simulink model "inter_machine_oscillation"  (R2014a)
settings: Solver=ode23tb  StartTime=0.0  StopTime=10  MaxStep=1/60  RelTol=1e-4
StartFcn:
  | tic;
StopFcn:
  | toc;
libraries: powerlib x6, simulink x2
settings Model: Creator=gdudgeon  LastModifiedBy=cosorio
settings DataIOCC: SaveOutput=off  DSMLogging=off  SaveTime=off
settings OptimizationCC: ExpressionDepthLimit=2147483647
settings DebuggingCC: UnderspecifiedInitializationDetection=Classic  FcnCallInpInsideContextMsg=UseLocalSettings  StateNameClashWarn=warning
settings GRTTargetCC: CombineOutputUpdateFcns=off  GRTInterface=on

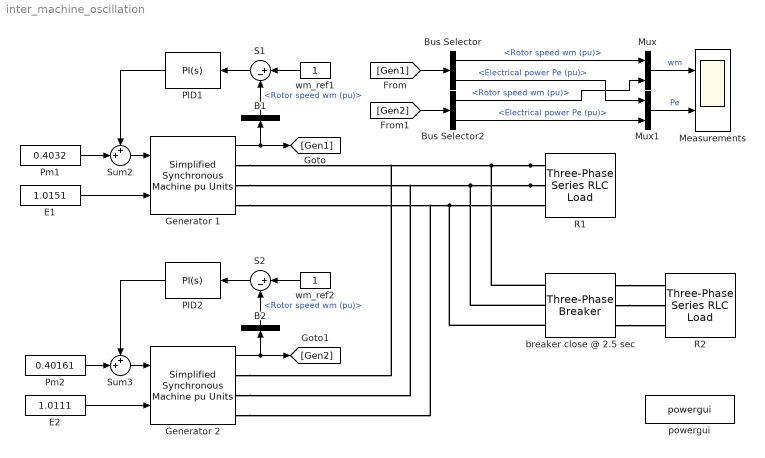
== system inter_machine_oscillation ==
  B1 : BusSelector  OutputSignals=Rotor speed wm (pu)
  B2 : BusSelector  OutputSignals=Rotor speed wm (pu)
  Bus Selector : BusSelector  OutputSignals=Rotor speed wm (pu),Electrical power Pe (pu)
  Bus Selector2 : BusSelector  OutputSignals=Rotor speed wm (pu),Electrical power Pe (pu)
  E1 : Constant  Value=1.0151
  E2 : Constant  Value=1.0111
  Generator 1 : powerlib/Machines/Simplified Synchronous Machine pu Units  ConnectionType=3-wire Y  MechanicalLoad=Mechanical power Pm  MeasurementBus=off  NominalParameters=[5e6 6600 60]  Mechanical=[3.7 0 20]  InternalRL="[0.02  0.3]"  InitialConditions=[0 6.78897 0.4 0.4 0.4 0 -120 120]  Units=0  LoadFlowParameters=[1 2000040 0 0 0]  TsPowergui=0  TsBlock=-1  BusType=PQ  Pref=2e6  Qref=0  Qmin=-inf  Qmax=+inf  PLF=0  QLF=0
      settings: AttributesFormatString=%<NominalParameters>
  Generator 2 : powerlib/Machines/Simplified Synchronous Machine pu Units  ConnectionType=3-wire Y  MechanicalLoad=Mechanical power Pm  MeasurementBus=off  NominalParameters=[5e6 6600 60]  Mechanical=[1.7 0 20]  InternalRL="[0.01  0.3]"  InitialConditions=[0 6.81591 0.400009 0.400009 0.400009 1.20401e-12 -120 120]  Units=0  LoadFlowParameters=[2 2000000 0 0 0]  TsPowergui=0  TsBlock=-1  BusType=swing  Pref=0  Qref=0  Qmin=-inf  Qmax=+inf  PLF=0  QLF=0
      settings: AttributesFormatString=%<NominalParameters>
  Measurements : Scope  NumInputPorts=2
      settings: YMin=0.8~0.25  YMax=1.1~0.75  SaveName=measurements
  Mux : Mux  Inputs=2
  Mux1 : Mux  Inputs=2
  PID1 : simulink/Continuous/PID Controller  Controller=PI  TimeDomain=Continuous-time  SampleTime=1  IntegratorMethod=Forward Euler  FilterMethod=Forward Euler  Form=Parallel  P=25  I=50  D=0  N=100  InitialConditionSource=internal  InitialConditionForIntegrator=0  InitialConditionForFilter=0  ExternalReset=none  LimitOutput=off  UpperSaturationLimit=2  LowerSaturationLimit=0  LinearizeAsGain=on  AntiWindupMode=none  Kb=1  TrackingMode=off  Kt=1  PParamMin=[]  PParamMax=[]  IParamMin=[]  IParamMax=[]  DParamMin=[]  DParamMax=[]  NParamMin=[]  NParamMax=[]  KbParamMin=[]  KbParamMax=[]  KtParamMin=[]  KtParamMax=[]  POutMin=[]  POutMax=[]  IOutMin=[]  IOutMax=[]  DOutMin=[]  DOutMax=[]  NOutMin=[]  NOutMax=[]  KbOutMin=[]  KbOutMax=[]  KtOutMin=[]  KtOutMax=[]  IntegratorOutMin=[]  IntegratorOutMax=[]  FilterOutMin=[]  FilterOutMax=[]  SumOutMin=[]  SumOutMax=[]  SumI1OutMin=[]  SumI1OutMax=[]  SumI2OutMin=[]  SumI2OutMax=[]  SumI3OutMin=[]  SumI3OutMax=[]  SumDOutMin=[]  SumDOutMax=[]  SaturationOutMin=[]  SaturationOutMax=[]  IntegratorContinuousStateAttributes=''  IntegratorStateMustResolveToSignalObject=off  IntegratorRTWStateStorageClass=Auto  FilterContinuousStateAttributes=''  FilterStateMustResolveToSignalObject=off  FilterRTWStateStorageClass=Auto
  PID2 : simulink/Continuous/PID Controller  Controller=PI  TimeDomain=Continuous-time  SampleTime=1  IntegratorMethod=Forward Euler  FilterMethod=Forward Euler  Form=Parallel  P=25  I=50  D=0  N=100  InitialConditionSource=internal  InitialConditionForIntegrator=0  InitialConditionForFilter=0  ExternalReset=none  LimitOutput=off  UpperSaturationLimit=2  LowerSaturationLimit=0  LinearizeAsGain=on  AntiWindupMode=none  Kb=1  TrackingMode=off  Kt=1  PParamMin=[]  PParamMax=[]  IParamMin=[]  IParamMax=[]  DParamMin=[]  DParamMax=[]  NParamMin=[]  NParamMax=[]  KbParamMin=[]  KbParamMax=[]  KtParamMin=[]  KtParamMax=[]  POutMin=[]  POutMax=[]  IOutMin=[]  IOutMax=[]  DOutMin=[]  DOutMax=[]  NOutMin=[]  NOutMax=[]  KbOutMin=[]  KbOutMax=[]  KtOutMin=[]  KtOutMax=[]  IntegratorOutMin=[]  IntegratorOutMax=[]  FilterOutMin=[]  FilterOutMax=[]  SumOutMin=[]  SumOutMax=[]  SumI1OutMin=[]  SumI1OutMax=[]  SumI2OutMin=[]  SumI2OutMax=[]  SumI3OutMin=[]  SumI3OutMax=[]  SumDOutMin=[]  SumDOutMax=[]  SaturationOutMin=[]  SaturationOutMax=[]  IntegratorContinuousStateAttributes=''  IntegratorStateMustResolveToSignalObject=off  IntegratorRTWStateStorageClass=Auto  FilterContinuousStateAttributes=''  FilterStateMustResolveToSignalObject=off  FilterRTWStateStorageClass=Auto
  Pm1 : Constant  Value=0.4032
  Pm2 : Constant  Value=0.40161
  R1 : powerlib/Elements/Three-Phase Series RLC Load  LConnTagsString=A|B|C  Configuration=Y (grounded)  NominalVoltage=6600  NominalFrequency=60  ActivePower=4e6  InductivePower=0  CapacitivePower=0  Measurements=None  LoadType=constant Z
      settings: AttributesFormatString=|
      | Vn = %<NominalVoltage> Vrms
      | P = %<ActivePower> W
  R2 : powerlib/Elements/Three-Phase Series RLC Load  LConnTagsString=A|B|C  Configuration=Y (grounded)  NominalVoltage=6600  NominalFrequency=60  ActivePower=1e6  InductivePower=0  CapacitivePower=0  Measurements=None  LoadType=constant Z
      settings: AttributesFormatString=|
      | Vn = %<NominalVoltage> Vrms
      | P = %<ActivePower> W
  S1 : Sum  Inputs=|+-
  S2 : Sum  Inputs=|+-
  Sum2 : Sum  Inputs=++|
  Sum3 : Sum  Inputs=++|
  breaker close @ 2.5 sec : powerlib/Elements/Three-Phase Breaker  InitialState=open  SwitchA=on  SwitchB=on  SwitchC=on  SwitchTimes=2.5  External=off  BreakerResistance=0.001  SnubberResistance=1e6  SnubberCapacitance=inf  Measurements=None
  powergui : powerlib/powergui  SimulationMode=Continuous  SolverType=Tustin  SampleTime=1e-4  frequency=60  SPID=off  DisableSnubberDevices=off  DisableRonSwitches=off  DisableVfSwitches=off  SwTol=0  Interpol=off  DisplayEquations=off  Ts=0  methode=off  frequencyindice=60  Pbase=100e6  ErrMax=0.0001  Iterations=50  UnitsV=kV  UnitsW=MW  FunctionMessages=off  echomessages=off  HookPort=off  EnableUseOfTLC=off  x0status=blocks  RestoreLinks=warning  ResistiveCurrentMeasurement=off  Frange=[0:2:500]  Ylog=off  Xlog=on  ShowGrid=off  save=off  variable=ZData  structure=0  ZoomFFT=on  StartTime=0.0  cycles=1  DisplayStyle=1  fundamental=60  FreqAxis=off  MaxFrequency=1000  frequencyindicesteady=1  RmsSteady=1  display=off
  wm_ref1 : Constant
  wm_ref2 : Constant
  wires:
  E1/1 -> Generator 1/2
  E2/1 -> Generator 2/2
  Generator 1/1 -> [Gen1], B1/1
  Generator 2/1 -> [Gen2], B2/1
  [Gen1] -> Bus Selector/1
  [Gen2] -> Bus Selector2/1
  Bus Selector2/2 -> Mux1/2  "<Electrical power Pe (pu)>"
  Bus Selector/1 -> Mux/1  "<Rotor speed wm (pu)>"
  Bus Selector2/1 -> Mux/2  "<Rotor speed wm (pu)>"
  Bus Selector/2 -> Mux1/1  "<Electrical power Pe (pu)>"
  Mux1/1 -> Measurements/2  "Pe"
  Mux/1 -> Measurements/1  "wm"
  B1/1 -> S1/2  "<Rotor speed wm (pu)>"
  S1/1 -> PID1/1
  PID1/1 -> Sum2/1
  wm_ref1/1 -> S1/1
  B2/1 -> S2/2  "<Rotor speed wm (pu)>"
  S2/1 -> PID2/1
  PID2/1 -> Sum3/1
  wm_ref2/1 -> S2/1
  Pm2/1 -> Sum3/2
  Sum3/1 -> Generator 2/1
  Pm1/1 -> Sum2/2
  Sum2/1 -> Generator 1/1
  connections:
  R1/LConn1 -- Generator 2/RConn1 -- Generator 1/RConn1 -- breaker close @ 2.5 sec/LConn1
  R1/LConn2 -- breaker close @ 2.5 sec/LConn2 -- Generator 2/RConn2 -- Generator 1/RConn2
  breaker close @ 2.5 sec/LConn3 -- R1/LConn3 -- Generator 1/RConn3 -- Generator 2/RConn3
  breaker close @ 2.5 sec/RConn1 -- R2/LConn1
  breaker close @ 2.5 sec/RConn2 -- R2/LConn2
  breaker close @ 2.5 sec/RConn3 -- R2/LConn3
